simulink model "V2GbidirectionalEV"  (R2019a)
settings: Solver=VariableStepAuto  StartTime=0.0  StopTime=1.5  RelTol=1e-3
undefined symbols (not defined in the file): Ion, Lithium
libraries: powerlib x28, simulink x2, electricdrivelib x1
settings Model: Creator=BPW  LastModifiedBy=BPW

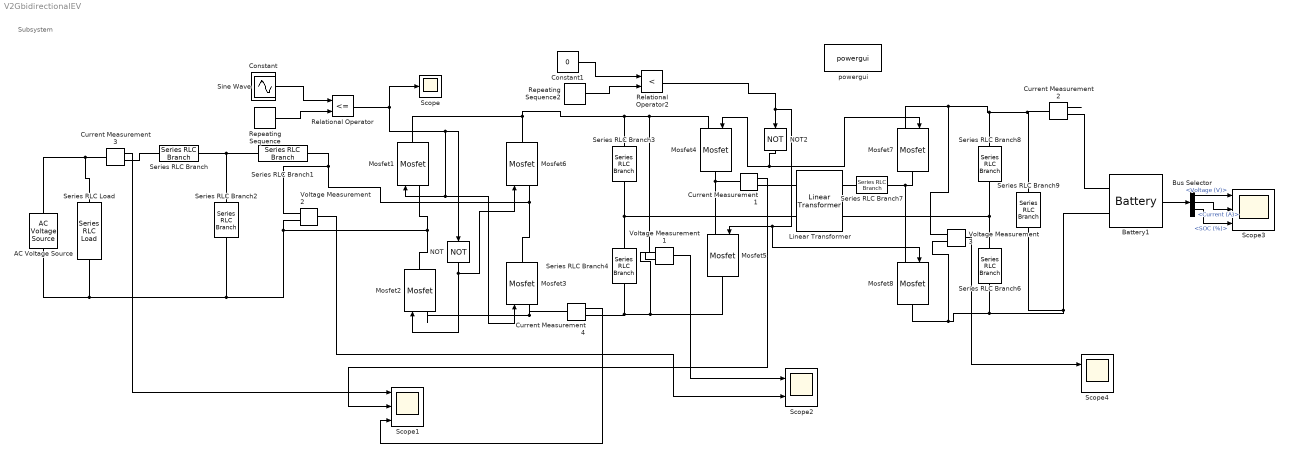
== system V2GbidirectionalEV ==
  note: Subsystem
  AC Voltage Source : powerlib/Electrical Sources/AC Voltage Source  Amplitude=220  Phase=0  Frequency=50  SampleTime=0  Measurements=None  BusType=swing  Pref=10e3  Qref=0  Qmin=-inf  Qmax=+inf
      settings: SourceProductName=Simscape Electrical
  Battery1 : electricdrivelib/Extra Sources/Battery  BatType=Lithium-Ion  ShowTempParam=off  ThermalPreset=no  ShowAgeParam=off  NomV=48  NomQ=5000  SOC=50  Batt_Tr=1  PresetModel=on  MaxQ=5000  MinV=36  FullV=55.8714  Dis_rate=2173.913  R=9.6e-05  Normal_OP=4521.7391  expZone="[51.85852      245.6522]"  current=[6.5 13 32.5]  Units=Time  Tci=20  NomT=20  T2=-30  MaxQ2=4.8  FullV2=7.1  Normal_OP2=5.655  expZone2="[6.58           1]"  Rca=0.6  ti=2000  Dp=0  Neq0=0  Tsim=1e6  Ta1=25  Qeol=5.4*0.9  Reol=0.013333*1.2  Char_age=[2.3478, 3]  Dis_age=[2.3478, 10]  N1=1500  N2=10500  N3=1000  N4=1400  Ta2=45  N5=950
      settings: SourceProductName=Simscape Electrical
  Bus Selector : BusSelector  OutputSignals=Voltage (V),Current (A),SOC (%)
  Constant : Constant  Value=0
  Constant1 : Constant  Value=0
  Current Measurement{1..4} (4 alike) : powerlib/Measurements/Current Measurement  PhasorSimulation=off  OutputType=Complex  PSBequivalent=0
      settings: SourceProductName=Simscape Electrical
  Linear Transformer : powerlib/Elements/Linear Transformer  UNITS=pu  NominalPower=[ 2500 1000 ]  winding1="[ 2  0  0.008 ]"  winding2="[24  0  0.0008 ]"  ThreeWindings=off  winding3=[ 315e3 0.002 0.08 ]  RmLm=[ 50000 50000 ]  Measurements=None  DataType=off
      settings: SourceProductName=Simscape Electrical
  Mosfet{1..8} (8 alike) : powerlib/Power Electronics/Mosfet  Ron=0.1  Lon=0  Rd=0.01  Vfd=0  IC=0  Rs=1e5  Cs=inf  Measurements=off
      settings: SourceProductName=Simscape Electrical
  NOT : Logic  Operator=NOT  IconShape=distinctive  AllPortsSameDT=off  OutDataTypeStr=boolean
  NOT2 : Logic  Operator=NOT  IconShape=distinctive  AllPortsSameDT=off  OutDataTypeStr=boolean
  Relational Operator : RelationalOperator  Operator=<=  OutDataTypeStr=boolean  RndMeth=Simplest
  Relational Operator2 : RelationalOperator  Operator=<  OutDataTypeStr=boolean  RndMeth=Simplest
  Repeating Sequence : simulink/Sources/Repeating Sequence  rep_seq_t=[0 1e-3]  rep_seq_y=[-1 1]
  Repeating Sequence2 : simulink/Sources/Repeating Sequence  rep_seq_t=[0 20e-3]  rep_seq_y=[-1 1]
  Scope : Scope
  Scope1 : Scope  NumInputPorts=3
  Scope2 : Scope  NumInputPorts=2
  Scope3 : Scope  NumInputPorts=3
  Scope4 : Scope  NumInputPorts=2
  Series RLC Branch : powerlib/Elements/Series RLC Branch  LConnTagsString=__new0  RConnTagsString=__new0  BranchType=L  Resistance=1  Inductance=250e-6  SetiL0=off  InitialCurrent=0  Capacitance=1e-6  Setx0=off  InitialVoltage=0  Measurements=None
      settings: SourceProductName=Simscape Electrical
  Series RLC Branch1 : powerlib/Elements/Series RLC Branch  LConnTagsString=__new0  RConnTagsString=__new0  BranchType=L  Resistance=1  Inductance=250e-6  SetiL0=off  InitialCurrent=0  Capacitance=1e-6  Setx0=off  InitialVoltage=0  Measurements=None
      settings: SourceProductName=Simscape Electrical
  Series RLC Branch2 : powerlib/Elements/Series RLC Branch  LConnTagsString=__new0  RConnTagsString=__new0  BranchType=C  Resistance=1  Inductance=1e-3  SetiL0=off  InitialCurrent=0  Capacitance=600e-6  Setx0=off  InitialVoltage=0  Measurements=None
      settings: SourceProductName=Simscape Electrical
  Series RLC Branch3 : powerlib/Elements/Series RLC Branch  LConnTagsString=__new0  RConnTagsString=__new0  BranchType=C  Resistance=1  Inductance=1e-3  SetiL0=off  InitialCurrent=0  Capacitance=100e-6  Setx0=off  InitialVoltage=0  Measurements=None
      settings: SourceProductName=Simscape Electrical
  Series RLC Branch4 : powerlib/Elements/Series RLC Branch  LConnTagsString=__new0  RConnTagsString=__new0  BranchType=C  Resistance=1  Inductance=1e-3  SetiL0=off  InitialCurrent=0  Capacitance=100e-6  Setx0=off  InitialVoltage=0  Measurements=None
      settings: SourceProductName=Simscape Electrical
  Series RLC Branch6 : powerlib/Elements/Series RLC Branch  LConnTagsString=__new0  RConnTagsString=__new0  BranchType=C  Resistance=0.05  Inductance=1e-3  SetiL0=off  InitialCurrent=0  Capacitance=600e-6  Setx0=off  InitialVoltage=0  Measurements=None
      settings: SourceProductName=Simscape Electrical
  Series RLC Branch7 : powerlib/Elements/Series RLC Branch  LConnTagsString=__new0  RConnTagsString=__new0  BranchType=L  Resistance=1  Inductance=4.7e-6  SetiL0=off  InitialCurrent=0  Capacitance=1e-6  Setx0=off  InitialVoltage=0  Measurements=None
      settings: SourceProductName=Simscape Electrical
  Series RLC Branch8 : powerlib/Elements/Series RLC Branch  LConnTagsString=__new0  RConnTagsString=__new0  BranchType=C  Resistance=0.05  Inductance=1e-3  SetiL0=off  InitialCurrent=0  Capacitance=600e-6  Setx0=off  InitialVoltage=0  Measurements=None
      settings: SourceProductName=Simscape Electrical
  Series RLC Branch9 : powerlib/Elements/Series RLC Branch  LConnTagsString=__new0  RConnTagsString=__new0  BranchType=RC  Resistance=0.05  Inductance=1e-3  SetiL0=off  InitialCurrent=0  Capacitance=600e-6  Setx0=off  InitialVoltage=0  Measurements=None
      settings: SourceProductName=Simscape Electrical
  Series RLC Load : powerlib/Elements/Series RLC Load  LConnTagsString=a  RConnTagsString=__new0  NominalVoltage=220  NominalFrequency=50  ActivePower=10e3  InductivePower=100  CapacitivePower=100  Setx0=off  InitialVoltage=0  SetiL0=off  InitialCurrent=0  Measurements=None  LoadType=constant Z
      settings: SourceProductName=Simscape Electrical
  Sine Wave : Sin  Amplitude=0.8  Frequency=314  SampleTime=0
  Voltage Measurement1 : powerlib/Measurements/Voltage Measurement  PhasorSimulation=off  OutputType=Complex  PSBequivalent=0
      settings: SourceProductName=Simscape Electrical
  Voltage Measurement2 : powerlib/Measurements/Voltage Measurement  PhasorSimulation=off  OutputType=Complex  PSBequivalent=0
      settings: SourceProductName=Simscape Electrical
  Voltage Measurement3 : powerlib/Measurements/Voltage Measurement  PhasorSimulation=off  OutputType=Complex  PSBequivalent=0
      settings: SourceProductName=Simscape Electrical
  powergui : powerlib/powergui  Priority=1  SimulationMode=Discrete  SampleTime=1e-6  frequency=60  Iterations=50  frequencyindice=0  Pbase=100e6  ErrMax=1e-4  UnitsV=kV  UnitsW=MW  buscounter=0  FunctionMessages=off  echomessages=off  EnableUseOfTLC=off  CurrentSourceSwitches=off  DisableSnubberDevices=off  DisableRonSwitches=off  DisableVfSwitches=off  DisplayEquations=off  AutomaticDiscreteSolvers=off  SolverType=Tustin/Backward Euler (TBE)  Interpol=off  ExternalGateDelay=off  methode=off  Ts=100  x0status=blocks  SPID=on  SwTol=0  HookPort=off  NonlinearTolerance=0  nMaxIteration=15  ContinueOnMaxIteration=off  RestoreLinks=warning  ResistiveCurrentMeasurement=off  Frange=[0:2:500]  Ylog=off  Xlog=on  ShowGrid=off  save=off  variable=ZData  structure=0  ZoomFFT=off  StartTime=0.0  cycles=1  DisplayStyle=1  fundamental=60  FreqAxis=off  MaxFrequency=1000  frequencyindicesteady=1  RmsSteady=1  display=off
      settings: SourceProductName=Simscape Electrical
  wires:
  Current Measurement2/1 -> ?
  Voltage Measurement3/1 -> Scope4/1
  Constant/1 -> Relational Operator/1
  Voltage Measurement1/1 -> Scope2/1
  Current Measurement4/1 -> Scope1/3
  Battery1/1 -> Bus Selector/1
  Bus Selector/2 -> Scope3/2  "<Current (A)>"
  Constant1/1 -> Relational Operator2/1
  Current Measurement1/1 -> Scope1/2
  Relational Operator2/1 -> Mosfet8/1, Mosfet5/1, NOT2/1
  Repeating Sequence2/1 -> Relational Operator2/2
  Current Measurement3/1 -> Scope1/1
  NOT2/1 -> Mosfet7/1, Mosfet4/1
  Voltage Measurement2/1 -> Scope2/2
  NOT/1 -> Mosfet6/1, Mosfet2/1
  Repeating Sequence/1 -> Relational Operator/2
  Relational Operator/1 -> Scope/1, Mosfet1/1, Mosfet3/1, NOT/1
  Bus Selector/3 -> Scope3/3  "<SOC (%)>"
  Bus Selector/1 -> Scope3/1  "<Voltage (V)>"
  connections:
  Linear Transformer/RConn1 -- Series RLC Branch7/LConn1
  Battery1/LConn2 -- Series RLC Branch9/RConn1 -- Mosfet8/RConn1 -- Voltage Measurement3/LConn2 -- Series RLC Branch6/RConn1
  Current Measurement1/RConn1 -- Linear Transformer/LConn1
  Current Measurement2/LConn1 -- Series RLC Branch9/LConn1 -- Series RLC Branch8/LConn1 -- Voltage Measurement3/LConn1 -- Mosfet7/LConn1
  Mosfet2/LConn1 -- Current Measurement4/LConn1 -- Mosfet3/LConn1
  Mosfet1/RConn1 -- Mosfet4/LConn1 -- Voltage Measurement1/LConn2 -- Series RLC Branch3/LConn1 -- Mosfet6/RConn1
  Series RLC Branch1/RConn1 -- Mosfet3/RConn1 -- Mosfet6/LConn1 -- Voltage Measurement2/LConn1
  AC Voltage Source/RConn1 -- Series RLC Load/LConn1 -- Current Measurement3/LConn1
  Mosfet5/LConn1 -- Current Measurement1/LConn1 -- Mosfet4/RConn1
  Mosfet5/RConn1 -- Current Measurement4/RConn1 -- Series RLC Branch4/RConn1 -- Voltage Measurement1/LConn1
  Current Measurement2/RConn1 -- Battery1/LConn1
  Series RLC Branch1/LConn1 -- Series RLC Branch/RConn1 -- Series RLC Branch2/LConn1
  AC Voltage Source/LConn1 -- Series RLC Load/RConn1 -- Voltage Measurement2/LConn2 -- Mosfet1/LConn1 -- Mosfet2/RConn1 -- Series RLC Branch2/RConn1
  Linear Transformer/RConn2 -- Series RLC Branch6/LConn1 -- Series RLC Branch8/RConn1
  Series RLC Branch4/LConn1 -- Linear Transformer/LConn2 -- Series RLC Branch3/RConn1
  Series RLC Branch7/RConn1 -- Mosfet8/LConn1 -- Mosfet7/RConn1
  Current Measurement3/RConn1 -- Series RLC Branch/LConn1
